simulink model "umbral_adaptativo"  (R2018a)
settings: Solver=VariableStepAuto  StartTime=0.0  StopTime=10.0  RelTol=1e-3
values from neighbouring files (symbols this model uses):
  tao1 = 0.000002    (= 2e-06)    [nn_arx_prueba.m]
  tao2 = tao1    (= 2e-06)    [nn_arx_prueba.m]
  taod = 1    [nn_arx_prueba.m]
settings Model: Creator=carma  LastModifiedBy=carma

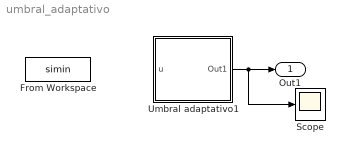
== system umbral_adaptativo ==
  From Workspace : FromWorkspace  VariableName=simin  SampleTime=0
  Scope : Scope
  Umbral adaptativo1 : Subsystem
  Out1 : Outport
  wires:
  Umbral adaptativo1/1(Out1) -> Scope/1, Out1/1

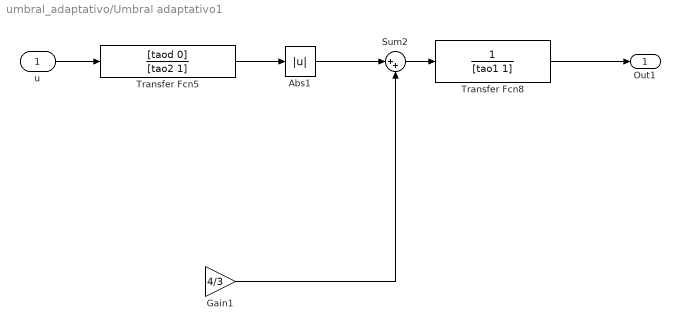
== system umbral_adaptativo/Umbral adaptativo1 ==
  u : Inport
  Abs1 : Abs
  Gain1 : Gain  Gain=4/3
  Sum2 : Sum  Inputs=|++
  Transfer Fcn5 : TransferFcn  Numerator=[taod 0]  Denominator=[tao2 1]
  Transfer Fcn8 : TransferFcn  Denominator=[tao1 1]
  Out1 : Outport
  wires:
  Gain1/1 -> Sum2/2
  Sum2/1 -> Transfer Fcn8/1
  Transfer Fcn8/1 -> Out1/1
  Transfer Fcn5/1 -> Abs1/1
  Abs1/1 -> Sum2/1
  u/1 -> Transfer Fcn5/1
